simulink model "sla_tffcn"  (R2015b)
settings: Solver=ode45  StartTime=0.0  StopTime=1  MaxStep=0.0001  RelTol=1e-3
PreLoadFcn:
  | La = 1e-3;      % 電機子インダクタンス [H]
  | Ra = 1;         % 電機子抵抗 [Ω]
  | Ke = 0.05;      % 逆起電力定数 [V/(rad/s)]
  | Kt = 0.05;      % トルク定数 [N*m/A]
  | J = 1e-4;       % ロータ慣性モーメント [kg*m^2]
  | B = 1e-6;       % ロータ動摩擦係数 [N*m/(rad/s)]
  | TL = 0;         % 負荷トルク [N*m]
  | sys = tf([0.015 0.38],[1 0.15]);
  | sysD = c2d(sys,1/1000, 'tustin');
  | [numd, dend] = tfdata(sysD,'v');
undefined symbols (not defined in the file or in its folder): dend, numd
settings Model: Creator=yyamamot  LastModifiedBy=amatsumo
settings DataIOCC: SaveFormat=Array  SignalLoggingSaveFormat=ModelDataLogs
settings OptimizationCC: BlockReduction=off  ConditionallyExecuteInputs=off  ExpressionDepthLimit=2147483647  OptimizeModelRefInitCode=on  LifeSpan=1
settings DebuggingCC: UnderspecifiedInitializationDetection=Classic  MergeDetectMultiDrivingBlocksExec=none  SolverPrmCheckMsg=warning  ParameterPrecisionLossMsg=none  ParameterTunabilityLossMsg=none  FcnCallInpInsideContextMsg=UseLocalSettings  StateNameClashWarn=warning
settings HardwareCC: ProdBitPerPointer=32  ProdLargestAtomicFloat=None  ProdIntDivRoundTo=Undefined  ProdEndianess=Unspecified  ProdWordSize=32  ProdHWDeviceType=32-bit Generic
settings RTWCC: SystemTargetFile=ert.tlc  GenCodeOnly=on  TemplateMakefile=ert_default_tmf  Description=Embedded Coder  GenerateReport=on  IncludeHyperlinkInReport=on  LaunchReport=on
settings CodeAppCC: IgnoreCustomStorageClasses=off  CustomSymbolStrType=$N$R$M  InternalIdentifier=Classic
settings ERTTargetCC: GenerateSampleERTMain=on  ERTCustomFileTemplate=example_file_process.tlc
settings ConfigComp: CovModelRefEnable=Off  CovSFcnEnable=off

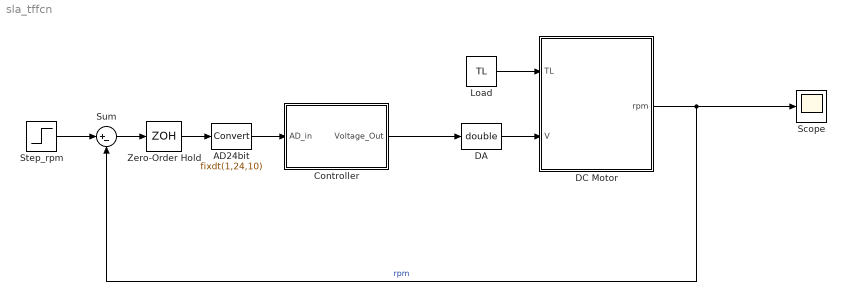
== system sla_tffcn ==
  AD24bit : DataTypeConversion  OutMin=-8000  OutMax=8000  OutDataTypeStr=fixdt(1,24,10)  SaturateOnIntegerOverflow=on
  Controller : Subsystem
  DA : DataTypeConversion  OutDataTypeStr=double
  DC Motor : Subsystem
  Load : Constant  Value=TL
  Scope : Scope
  Step_rpm : Step  Time=0.1  After=500  SampleTime=0
  Sum : Sum  Inputs=|+-
  Zero-Order Hold : ZeroOrderHold  SampleTime=1/1000
  wires:
  Load/1 -> DC Motor/1(TL)
  DC Motor/1(rpm) -> Scope/1, Sum/2  "rpm"
  Controller/1(Voltage_Out) -> DA/1
  Sum/1 -> Zero-Order Hold/1
  Step_rpm/1 -> Sum/1
  Zero-Order Hold/1 -> AD24bit/1
  DA/1 -> DC Motor/2(V)
  AD24bit/1 -> Controller/1(AD_in)

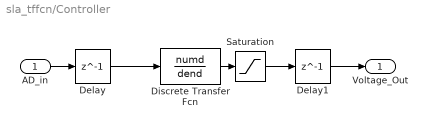
== system sla_tffcn/Controller ==
  AD_in : Inport
  Delay : Delay  DelayLength=1
  Delay1 : Delay  DelayLength=1
  Discrete Transfer Fcn : DiscreteTransferFcn  Numerator=numd  Denominator=dend  NumCoefMin=-1  NumCoefMax=1  DenCoefMin=-1  DenCoefMax=1  NumCoefDataTypeStr=fixdt(1,24,22)  DenCoefDataTypeStr=fixdt(1,24,22)  NumProductDataTypeStr=fixdt(1,48,32)  DenProductDataTypeStr=fixdt(1,48,32)  NumAccumDataTypeStr=fixdt(1,49,32)  DenAccumDataTypeStr=fixdt(1,49,32)  OutDataTypeStr=fixdt(1,49,32)  RndMeth=Nearest
  Saturation : Saturate  UpperLimit=20  LowerLimit=-20  OutMin=-20  OutMax=20  OutDataTypeStr=fixdt(1,24,18)
  Voltage_Out : Outport
  wires:
  AD_in/1 -> Delay/1
  Discrete Transfer Fcn/1 -> Saturation/1
  Saturation/1 -> Delay1/1
  Delay/1 -> Discrete Transfer Fcn/1
  Delay1/1 -> Voltage_Out/1

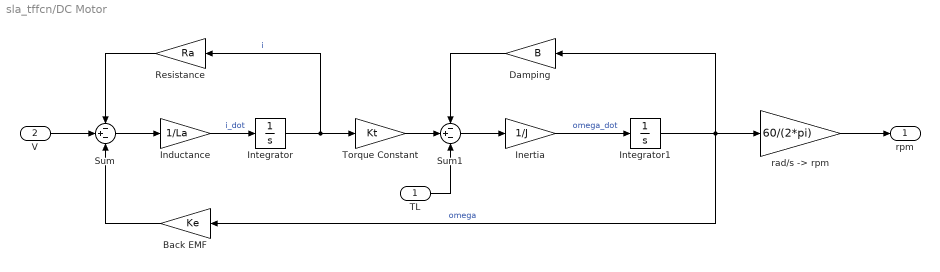
== system sla_tffcn/DC Motor ==
  TL : Inport
  V : Inport  Port=2
  Back EMF : Gain  Gain=Ke
  Damping : Gain  Gain=B
  Inductance : Gain  Gain=1/La
  Inertia : Gain  Gain=1/J
  Integrator : Integrator
  Integrator1 : Integrator
  Resistance : Gain  Gain=Ra
  Sum : Sum  Inputs=-+-
  Sum1 : Sum  Inputs=-+-
  Torque Constant : Gain  Gain=Kt
  "rad/s -> rpm" : Gain  Gain=60/(2*pi)
  rpm : Outport
  wires:
  Inductance/1 -> Integrator/1  "i_dot"
  Integrator/1 -> Resistance/1, Torque Constant/1  "i"
  Sum/1 -> Inductance/1
  Resistance/1 -> Sum/1
  Back EMF/1 -> Sum/3
  Torque Constant/1 -> Sum1/2
  Sum1/1 -> Inertia/1
  Inertia/1 -> Integrator1/1  "omega_dot"
  Integrator1/1 -> Damping/1, Back EMF/1, "rad/s -> rpm"/1  "omega"
  Damping/1 -> Sum1/1
  V/1 -> Sum/2
  TL/1 -> Sum1/3
  "rad/s -> rpm"/1 -> rpm/1
